simulink model "quadruped"  (R2019b)
settings: Solver=ode23t  StartTime=0.0  StopTime=Ts  RelTol=1e-3
values from neighbouring files (symbols this model uses):
  isdone = Isdone    [RL_reward.m]
  plane = [5, 50, 0.03]    [quadruped_sim_param.m]
  reward = Reward    [RL_reward.m]
  robot = Robot    [quadruped_sim_param.m]
undefined symbols (not defined in the file or in its folder): X, Y, Z
libraries: sm_lib x166, nesl_utility x90, simulink x33, rllib x1
(part 4 of 6)

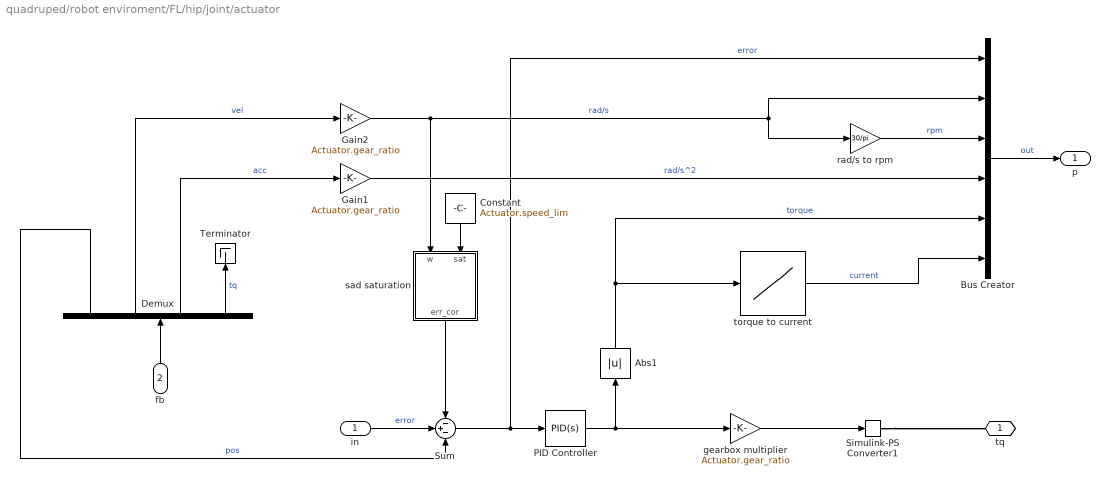
== system quadruped/robot enviroment/FL/hip/joint/actuator ==
  in : Inport
  fb : Inport  Port=2
  Abs1 : Abs
  Bus Creator : BusCreator  Inputs=6
  Constant : Constant  Value=Actuator.speed_lim
  Demux : Demux
  Gain1 : Gain  Gain=Actuator.gear_ratio
  Gain2 : Gain  Gain=Actuator.gear_ratio
  PID Controller : simulink/Continuous/PID Controller  Controller=PID  Form=Ideal  TimeDomain=Continuous-time  SampleTime=-1  IntegratorMethod=Forward Euler  FilterMethod=Forward Euler  ControllerParametersSource=internal  P=Actuator.Kp * pi / 180  I=Actuator.Ki  D=Actuator.Kd  UseFilter=on  N=Actuator.N  TunerSelectOption=Transfer Function Based (PID Tuner App)  InitialConditionSource=internal  InitialConditionForIntegrator=0  InitialConditionForFilter=0  DifferentiatorICPrevScaledInput=0  ExternalReset=none  TrackingMode=off  Kt=1  LimitOutput=on  UpperSaturationLimit=Actuator.torque_lim  LowerSaturationLimit=-Actuator.torque_lim  LinearizeAsGain=on  AntiWindupMode=none  Kb=1  POutMin=[]  POutMax=[]  IOutMin=[]  IOutMax=[]  DOutMin=[]  DOutMax=[]  NOutMin=[]  NOutMax=[]  SumOutMin=[]  SumOutMax=[]  SaturationOutMin=[]  SaturationOutMax=[]  PParamMin=[]  PParamMax=[]  IParamMin=[]  IParamMax=[]  DParamMin=[]  DParamMax=[]  NParamMin=[]  NParamMax=[]  KbParamMin=[]  KbParamMax=[]  KtParamMin=[]  KtParamMax=[]  KbOutMin=[]  KbOutMax=[]  KtOutMin=[]  KtOutMax=[]  IntegratorOutMin=[]  IntegratorOutMax=[]  FilterOutMin=[]  FilterOutMax=[]  SumI1OutMin=[]  SumI1OutMax=[]  SumI2OutMin=[]  SumI2OutMax=[]  SumI3OutMin=[]  SumI3OutMax=[]  SumI4OutMin=[]  SumI4OutMax=[]  SumDOutMin=[]  SumDOutMax=[]  DifferentiatorOutMin=[]  DifferentiatorOutMax=[]  FilterDiffOutCoefMin=[]  FilterDiffOutCoefMax=[]  ReciprocalOutMin=[]  ReciprocalOutMax=[]  SumDenOutMin=[]  SumDenOutMax=[]  SumNumOutMin=[]  SumNumOutMax=[]  DivideOutMin=[]  DivideOutMax=[]  IntegratorContinuousStateAttributes=''  IntegratorStateMustResolveToSignalObject=off  IntegratorRTWStateStorageClass=Auto  FilterContinuousStateAttributes=''  FilterStateMustResolveToSignalObject=off  FilterRTWStateStorageClass=Auto  ParallelPVariant=Passthrough  IdealPVariant=InternalParameters  IVariant=InternalParameters  DVariant=InternalParameters  IntegratorVariant=Continuous  SatVariant=Enabled  AWVariant=Passthrough  PCopyVariant=Disabled  TRVariant=Disabled  FdbkBlocksVariant=Forward  IdealPFdbkVariant=Disabled  SatFdbkVariant=Disabled  DerivativeFilterVariant=ContFilter  NVariant=InternalParameters  NCopyVariant=Disabled  FilterICVariant=InternalICsFilter  IntegratorICVariant=InternalICs  ExternalResetVariant=Disabled  TRSumVariant=Passthrough  SumFdbkVariant=Disabled  SumVariant=Sum_PID
  Simulink-PS Converter1 : nesl_utility/Simulink-PS Converter  PhysicalDomain=network_engine_domain  SubClassName=ps_input  LeftPortType=input  RightPortType=output  PseudoPeriodic=off  Frequencies=[]  NoiseDistribution=none  NoiseParameters=[]  Unit=N*m  AffineConversion=off  FilteringAndDerivatives=provide  SimscapeFilterOrder=1  InputFilterTimeConstant=0.001  UdotUserProvided=0
  Sum : Sum  Inputs=-+-
  Terminator : Terminator
  gearbox multiplier : Gain  Gain=Actuator.gear_ratio
  rad/s to rpm : Gain  Gain=30/pi
  sad saturation : Subsystem
  torque to current : Lookup_n-D  NumberOfTableDimensions=1  BreakpointsForDimension1=Actuator.torque_to_current(1,:)  Table=Actuator.torque_to_current(2,:)  InternalRulePriority=Speed  RndMeth=Simplest  InputSameDT=on
  tq : PMIOPort  Side=Right
  p : Outport
  wires:
  rad/s to rpm/1 -> Bus Creator/3  "rpm"
  Bus Creator/1 -> p/1  "out"
  torque to current/1 -> Bus Creator/6  "current"
  Sum/1 -> PID Controller/1, Bus Creator/1  "error"
  in/1 -> Sum/2  "error"
  Abs1/1 -> Bus Creator/5, torque to current/1  "torque"
  PID Controller/1 -> gearbox multiplier/1, Abs1/1
  gearbox multiplier/1 -> Simulink-PS Converter1/1
  Gain2/1 -> rad/s to rpm/1, Bus Creator/2, sad saturation/1(w)  "rad/s"
  fb/1 -> Demux/1
  Demux/1 -> Sum/3  "pos"
  Demux/2 -> Gain2/1  "vel"
  Demux/3 -> Gain1/1  "acc"
  Demux/4 -> Terminator/1  "tq"
  Gain1/1 -> Bus Creator/4  "rad/s^2"
  sad saturation/1(err_cor) -> Sum/1
  Constant/1 -> sad saturation/2(sat)
  connections:
  Simulink-PS Converter1/RConn1 -- tq/RConn1

== system quadruped/robot enviroment/FL/hip/joint/motor inertia ==
  Common Gear Constraint : sm_lib/Gears and Couplings/Gears/Common Gear Constraint  GearType=External  SpecificationType=CenterDistanceRatio  CenterDistance=0.5  CenterDistanceUnits=mm  GearRatio=Joint.actuator.gear_ratio  BaseGearRadius=10.0  BaseGearRadiusUnits=cm  FollGearRadius=10.0  FollGearRadiusUnits=cm  AssemblyGearRotation=Free
      settings: SourceProductName=Simscape Multibody  SourceProductBaseCode=MS
  Cylindrical Solid : sm_lib/Body Elements/Cylindrical Solid  GraphicAmbientColor=[0.15 0.15 0.15 1.0]  BasedOnType=Density  CenterOfMass=[0 0 0]  CenterOfMassUnits=m  GraphicDiffuseColor=[0.5 0.5 0.5]  CylinderLength=0.01  CylinderLengthUnits=m  CylinderRadius=0.01  CylinderRadiusUnits=m  Density=1000  DensityUnits=kg/m^3  DoExposeReferenceFrame=on  GraphicEmissiveColor=[0.0 0.0 0.0 1.0]  ExportEntireGeometry=off  SerializedFrames=<Frames/>  MarkerShape=Sphere  MarkerSize=10  GraphicType=FromGeometry  InertiaType=Custom  Mass=0  MassUnits=kg  MomentsOfInertia=[0 0 Joint.actuator.motor_inertia]  MomentsOfInertiaUnits=g*cm^2  GraphicOpacity=0  ProductsOfInertia=[0 0 0]  ProductsOfInertiaUnits=kg*m^2  GraphicShininess=75  GraphicSpecularColor=[0.5 0.5 0.5 1.0]  GraphicVisPropType=SimpleVisualProperties
  Revolute Joint1 : sm_lib/Joints/Revolute Joint  JointMode=Normal  SenseConstraintForce=off  SenseConstraintForceX=off  SenseConstraintForceY=off  SenseConstraintForceZ=off  SenseConstraintTorque=off  SenseConstraintTorqueX=off  SenseConstraintTorqueY=off  SenseConstraintTorqueZ=off  SenseTotalForce=off  SenseTotalForceX=off  SenseTotalForceY=off  SenseTotalForceZ=off  SenseTotalTorque=off  SenseTotalTorqueX=off  SenseTotalTorqueY=off  SenseTotalTorqueZ=off  CompositeWrenchDir=FollowerOnBase  CompositeWrenchFrame=BaseFrame  EquilibriumPosition=0  EquilibriumPositionUnits=deg  SpringStiffness=0  SpringStiffnessUnits=N*m/deg  DampingCoefficient=0  DampingCoefficientUnits=N*m/(deg/s)  TorqueActuationMode=NoTorque  MotionActuationMode=ComputedMotion  SensePosition=off  SenseVelocity=off  SenseAcceleration=off  SenseTorqueForce=off  SenseLowerLimitTorqueForce=off  SenseUpperLimitTorqueForce=off  LowerLimitSpecify=off  LowerLimitBound=-90  LowerLimitBoundUnits=deg  LowerLimitStiffness=1e4  LowerLimitStiffnessUnits=N*m/deg  LowerLimitDamping=10  LowerLimitDampingUnits=N*m/(deg/s)  LowerLimitTransitionRegionWidth=0.1  LowerLimitTransitionRegionWidthUnits=deg  UpperLimitSpecify=off  UpperLimitBound=90  UpperLimitBoundUnits=deg  UpperLimitStiffness=1e4  UpperLimitStiffnessUnits=N*m/deg  UpperLimitDamping=10  UpperLimitDampingUnits=N*m/(deg/s)  UpperLimitTransitionRegionWidth=0.1  UpperLimitTransitionRegionWidthUnits=deg  PositionTargetSpecify=off  PositionTargetPriority=High  PositionTargetValue=0  PositionTargetValueUnits=deg  VelocityTargetSpecify=off  VelocityTargetPriority=High  VelocityTargetValue=0  VelocityTargetValueUnits=deg/s
  Rigid Transform : sm_lib/Frames and Transforms/Rigid Transform  TranslationMethod=StandardAxis  TranslationStandardOffset=0.5  TranslationLengthUnit=mm  TranslationStandardAxis=+X  TranslationCartesianOffset=[0 0 0]  TranslationROffset=0  TranslationROffsetUnits=m  TranslationZOffset=0  TranslationZOffsetUnits=m  TranslationThetaOffset=0  TranslationThetaOffsetUnits=deg  RotationMethod=None  RotationAngleUnits=deg  RotationStandardAxis=+Z  RotationAngle=0.0  RotationArbitraryAxis=[0 0 1]  FollAlignAxisA=+X  BaseAlignAxisA=+Y  FollAlignAxisB=+Y  BaseAlignAxisB=+Z  RotationSequenceAxes=FollowerAxes  RotationSequence=XYX  RotationSequenceAngles=[0 0 0]  RotationSequenceAnglesUnits=deg  RotationMatrix=[1 0 0; 0 1 0; 0 0 1]
  B : PMIOPort  Side=Right
  F : PMIOPort  Port=2  Side=Left
  connections:
  Revolute Joint1/LConn1 -- Cylindrical Solid/RConn1 -- Common Gear Constraint/LConn1
  Rigid Transform/LConn1 -- Revolute Joint1/RConn1
  Common Gear Constraint/RConn1 -- F/RConn1
  B/RConn1 -- Rigid Transform/RConn1

== system quadruped/robot enviroment/FL/leg/lower joint/joint ==
  in : Inport
  Abs1 : Abs
  Bus Creator1 : BusCreator  Inputs=4
  Bus Creator2 : BusCreator  Inputs=3
  "Hip joint " : sm_lib/Joints/Revolute Joint  JointMode=Normal  SenseConstraintForce=off  SenseConstraintForceX=off  SenseConstraintForceY=off  SenseConstraintForceZ=off  SenseConstraintTorque=off  SenseConstraintTorqueX=off  SenseConstraintTorqueY=off  SenseConstraintTorqueZ=off  SenseTotalForce=off  SenseTotalForceX=off  SenseTotalForceY=off  SenseTotalForceZ=off  SenseTotalTorque=off  SenseTotalTorqueX=off  SenseTotalTorqueY=off  SenseTotalTorqueZ=off  CompositeWrenchDir=FollowerOnBase  CompositeWrenchFrame=BaseFrame  EquilibriumPosition=0  EquilibriumPositionUnits=rad  SpringStiffness=Joint.stiffness  SpringStiffnessUnits=N*m/deg  DampingCoefficient=Joint.damping  DampingCoefficientUnits=N*m/(deg/s)  TorqueActuationMode=InputTorque  MotionActuationMode=ComputedMotion  SensePosition=on  SenseVelocity=on  SenseAcceleration=on  SenseTorqueForce=on  SenseLowerLimitTorqueForce=off  SenseUpperLimitTorqueForce=off  LowerLimitSpecify=off  LowerLimitBound=-90  LowerLimitBoundUnits=deg  LowerLimitStiffness=1e4  LowerLimitStiffnessUnits=N*m/deg  LowerLimitDamping=10  LowerLimitDampingUnits=N*m/(deg/s)  LowerLimitTransitionRegionWidth=0.1  LowerLimitTransitionRegionWidthUnits=deg  UpperLimitSpecify=off  UpperLimitBound=90  UpperLimitBoundUnits=deg  UpperLimitStiffness=1e4  UpperLimitStiffnessUnits=N*m/deg  UpperLimitDamping=10  UpperLimitDampingUnits=N*m/(deg/s)  UpperLimitTransitionRegionWidth=0.1  UpperLimitTransitionRegionWidthUnits=deg  PositionTargetSpecify=on  PositionTargetPriority=High  PositionTargetValue=Joint.base_angle  PositionTargetValueUnits=rad  VelocityTargetSpecify=off  VelocityTargetPriority=High  VelocityTargetValue=0  VelocityTargetValueUnits=deg/s
  PS-Simulink Converter{3..6} (4 alike) : nesl_utility/PS-Simulink Converter  PhysicalDomain=network_engine_domain  SubClassName=ps_output  LeftPortType=input  RightPortType=output  PseudoPeriodic=off  Frequencies=[]  Unit=inherit  AffineConversion=off
  actuator : Subsystem  mask{Actuator=Joint.actuator}
  motor inertia : Subsystem
  B : PMIOPort  Side=Left
  F : PMIOPort  Port=2  Side=Right
  p : Outport
  wires:
  PS-Simulink Converter5/1 -> Bus Creator1/3  "b"
  PS-Simulink Converter6/1 -> Abs1/1, Bus Creator1/4  "t"
  PS-Simulink Converter3/1 -> Bus Creator1/2  "w"
  in/1 -> actuator/1(in)
  Bus Creator1/1 -> actuator/2(fb)
  actuator/1(p) -> Bus Creator2/3  "actuator"
  Bus Creator2/1 -> p/1
  Abs1/1 -> Bus Creator2/2  "joint torque"
  PS-Simulink Converter4/1 -> Bus Creator2/1, Bus Creator1/1  "position"
  connections:
  "Hip joint "/RConn4 -- PS-Simulink Converter5/LConn1
  motor inertia/RConn1 -- "Hip joint "/LConn1 -- B/RConn1
  actuator/RConn1 -- "Hip joint "/LConn2
  "Hip joint "/RConn5 -- PS-Simulink Converter6/LConn1
  "Hip joint "/RConn2 -- PS-Simulink Converter4/LConn1
  "Hip joint "/RConn1 -- motor inertia/LConn1 -- F/RConn1
  "Hip joint "/RConn3 -- PS-Simulink Converter3/LConn1

== system quadruped/robot enviroment/FL/leg/upper joint/joint ==
  in : Inport
  Abs1 : Abs
  Bus Creator1 : BusCreator  Inputs=4
  Bus Creator2 : BusCreator  Inputs=3
  "Hip joint " : sm_lib/Joints/Revolute Joint  JointMode=Normal  SenseConstraintForce=off  SenseConstraintForceX=off  SenseConstraintForceY=off  SenseConstraintForceZ=off  SenseConstraintTorque=off  SenseConstraintTorqueX=off  SenseConstraintTorqueY=off  SenseConstraintTorqueZ=off  SenseTotalForce=off  SenseTotalForceX=off  SenseTotalForceY=off  SenseTotalForceZ=off  SenseTotalTorque=off  SenseTotalTorqueX=off  SenseTotalTorqueY=off  SenseTotalTorqueZ=off  CompositeWrenchDir=FollowerOnBase  CompositeWrenchFrame=BaseFrame  EquilibriumPosition=0  EquilibriumPositionUnits=rad  SpringStiffness=Joint.stiffness  SpringStiffnessUnits=N*m/deg  DampingCoefficient=Joint.damping  DampingCoefficientUnits=N*m/(deg/s)  TorqueActuationMode=InputTorque  MotionActuationMode=ComputedMotion  SensePosition=on  SenseVelocity=on  SenseAcceleration=on  SenseTorqueForce=on  SenseLowerLimitTorqueForce=off  SenseUpperLimitTorqueForce=off  LowerLimitSpecify=off  LowerLimitBound=-90  LowerLimitBoundUnits=deg  LowerLimitStiffness=1e4  LowerLimitStiffnessUnits=N*m/deg  LowerLimitDamping=10  LowerLimitDampingUnits=N*m/(deg/s)  LowerLimitTransitionRegionWidth=0.1  LowerLimitTransitionRegionWidthUnits=deg  UpperLimitSpecify=off  UpperLimitBound=90  UpperLimitBoundUnits=deg  UpperLimitStiffness=1e4  UpperLimitStiffnessUnits=N*m/deg  UpperLimitDamping=10  UpperLimitDampingUnits=N*m/(deg/s)  UpperLimitTransitionRegionWidth=0.1  UpperLimitTransitionRegionWidthUnits=deg  PositionTargetSpecify=on  PositionTargetPriority=High  PositionTargetValue=Joint.base_angle  PositionTargetValueUnits=rad  VelocityTargetSpecify=off  VelocityTargetPriority=High  VelocityTargetValue=0  VelocityTargetValueUnits=deg/s
  PS-Simulink Converter{3..6} (4 alike) : nesl_utility/PS-Simulink Converter  PhysicalDomain=network_engine_domain  SubClassName=ps_output  LeftPortType=input  RightPortType=output  PseudoPeriodic=off  Frequencies=[]  Unit=inherit  AffineConversion=off
  actuator : Subsystem  mask{Actuator=Joint.actuator}
  motor inertia : Subsystem
  B : PMIOPort  Side=Left
  F : PMIOPort  Port=2  Side=Right
  p : Outport
  wires:
  PS-Simulink Converter5/1 -> Bus Creator1/3  "b"
  PS-Simulink Converter6/1 -> Abs1/1, Bus Creator1/4  "t"
  PS-Simulink Converter3/1 -> Bus Creator1/2  "w"
  in/1 -> actuator/1(in)
  Bus Creator1/1 -> actuator/2(fb)
  actuator/1(p) -> Bus Creator2/3  "actuator"
  Bus Creator2/1 -> p/1
  Abs1/1 -> Bus Creator2/2  "joint torque"
  PS-Simulink Converter4/1 -> Bus Creator2/1, Bus Creator1/1  "position"
  connections:
  "Hip joint "/RConn4 -- PS-Simulink Converter5/LConn1
  motor inertia/RConn1 -- "Hip joint "/LConn1 -- B/RConn1
  actuator/RConn1 -- "Hip joint "/LConn2
  "Hip joint "/RConn5 -- PS-Simulink Converter6/LConn1
  "Hip joint "/RConn2 -- PS-Simulink Converter4/LConn1
  "Hip joint "/RConn1 -- motor inertia/LConn1 -- F/RConn1
  "Hip joint "/RConn3 -- PS-Simulink Converter3/LConn1

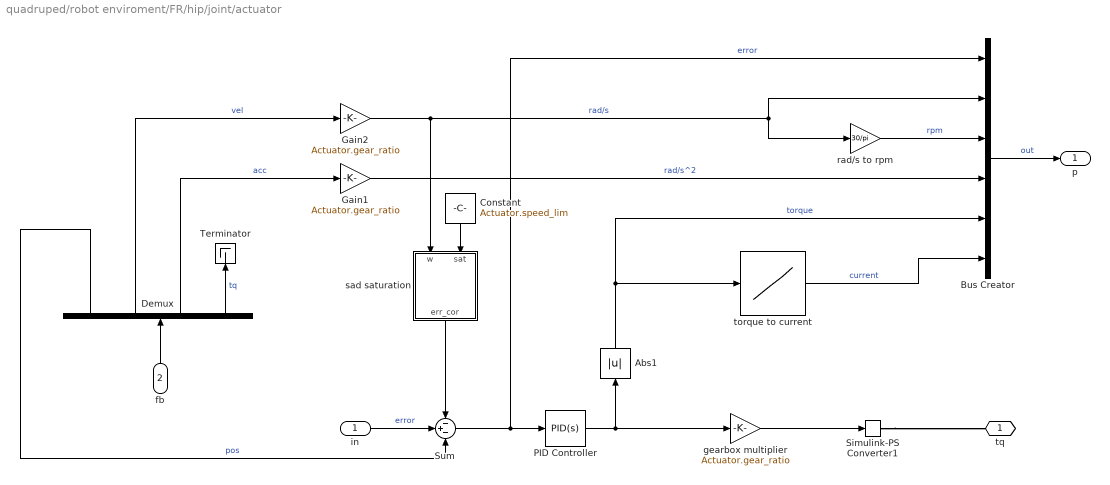
== system quadruped/robot enviroment/FR/hip/joint/actuator ==
  in : Inport
  fb : Inport  Port=2
  Abs1 : Abs
  Bus Creator : BusCreator  Inputs=6
  Constant : Constant  Value=Actuator.speed_lim
  Demux : Demux
  Gain1 : Gain  Gain=Actuator.gear_ratio
  Gain2 : Gain  Gain=Actuator.gear_ratio
  PID Controller : simulink/Continuous/PID Controller  Controller=PID  Form=Ideal  TimeDomain=Continuous-time  SampleTime=-1  IntegratorMethod=Forward Euler  FilterMethod=Forward Euler  ControllerParametersSource=internal  P=Actuator.Kp * pi / 180  I=Actuator.Ki  D=Actuator.Kd  UseFilter=on  N=Actuator.N  TunerSelectOption=Transfer Function Based (PID Tuner App)  InitialConditionSource=internal  InitialConditionForIntegrator=0  InitialConditionForFilter=0  DifferentiatorICPrevScaledInput=0  ExternalReset=none  TrackingMode=off  Kt=1  LimitOutput=on  UpperSaturationLimit=Actuator.torque_lim  LowerSaturationLimit=-Actuator.torque_lim  LinearizeAsGain=on  AntiWindupMode=none  Kb=1  POutMin=[]  POutMax=[]  IOutMin=[]  IOutMax=[]  DOutMin=[]  DOutMax=[]  NOutMin=[]  NOutMax=[]  SumOutMin=[]  SumOutMax=[]  SaturationOutMin=[]  SaturationOutMax=[]  PParamMin=[]  PParamMax=[]  IParamMin=[]  IParamMax=[]  DParamMin=[]  DParamMax=[]  NParamMin=[]  NParamMax=[]  KbParamMin=[]  KbParamMax=[]  KtParamMin=[]  KtParamMax=[]  KbOutMin=[]  KbOutMax=[]  KtOutMin=[]  KtOutMax=[]  IntegratorOutMin=[]  IntegratorOutMax=[]  FilterOutMin=[]  FilterOutMax=[]  SumI1OutMin=[]  SumI1OutMax=[]  SumI2OutMin=[]  SumI2OutMax=[]  SumI3OutMin=[]  SumI3OutMax=[]  SumI4OutMin=[]  SumI4OutMax=[]  SumDOutMin=[]  SumDOutMax=[]  DifferentiatorOutMin=[]  DifferentiatorOutMax=[]  FilterDiffOutCoefMin=[]  FilterDiffOutCoefMax=[]  ReciprocalOutMin=[]  ReciprocalOutMax=[]  SumDenOutMin=[]  SumDenOutMax=[]  SumNumOutMin=[]  SumNumOutMax=[]  DivideOutMin=[]  DivideOutMax=[]  IntegratorContinuousStateAttributes=''  IntegratorStateMustResolveToSignalObject=off  IntegratorRTWStateStorageClass=Auto  FilterContinuousStateAttributes=''  FilterStateMustResolveToSignalObject=off  FilterRTWStateStorageClass=Auto  ParallelPVariant=Passthrough  IdealPVariant=InternalParameters  IVariant=InternalParameters  DVariant=InternalParameters  IntegratorVariant=Continuous  SatVariant=Enabled  AWVariant=Passthrough  PCopyVariant=Disabled  TRVariant=Disabled  FdbkBlocksVariant=Forward  IdealPFdbkVariant=Disabled  SatFdbkVariant=Disabled  DerivativeFilterVariant=ContFilter  NVariant=InternalParameters  NCopyVariant=Disabled  FilterICVariant=InternalICsFilter  IntegratorICVariant=InternalICs  ExternalResetVariant=Disabled  TRSumVariant=Passthrough  SumFdbkVariant=Disabled  SumVariant=Sum_PID
  Simulink-PS Converter1 : nesl_utility/Simulink-PS Converter  PhysicalDomain=network_engine_domain  SubClassName=ps_input  LeftPortType=input  RightPortType=output  PseudoPeriodic=off  Frequencies=[]  NoiseDistribution=none  NoiseParameters=[]  Unit=N*m  AffineConversion=off  FilteringAndDerivatives=provide  SimscapeFilterOrder=1  InputFilterTimeConstant=0.001  UdotUserProvided=0
  Sum : Sum  Inputs=-+-
  Terminator : Terminator
  gearbox multiplier : Gain  Gain=Actuator.gear_ratio
  rad/s to rpm : Gain  Gain=30/pi
  sad saturation : Subsystem
  torque to current : Lookup_n-D  NumberOfTableDimensions=1  BreakpointsForDimension1=Actuator.torque_to_current(1,:)  Table=Actuator.torque_to_current(2,:)  InternalRulePriority=Speed  RndMeth=Simplest  InputSameDT=on
  tq : PMIOPort  Side=Right
  p : Outport
  wires:
  rad/s to rpm/1 -> Bus Creator/3  "rpm"
  Bus Creator/1 -> p/1  "out"
  torque to current/1 -> Bus Creator/6  "current"
  Sum/1 -> PID Controller/1, Bus Creator/1  "error"
  in/1 -> Sum/2  "error"
  Abs1/1 -> Bus Creator/5, torque to current/1  "torque"
  PID Controller/1 -> gearbox multiplier/1, Abs1/1
  gearbox multiplier/1 -> Simulink-PS Converter1/1
  Gain2/1 -> rad/s to rpm/1, Bus Creator/2, sad saturation/1(w)  "rad/s"
  fb/1 -> Demux/1
  Demux/1 -> Sum/3  "pos"
  Demux/2 -> Gain2/1  "vel"
  Demux/3 -> Gain1/1  "acc"
  Demux/4 -> Terminator/1  "tq"
  Gain1/1 -> Bus Creator/4  "rad/s^2"
  sad saturation/1(err_cor) -> Sum/1
  Constant/1 -> sad saturation/2(sat)
  connections:
  Simulink-PS Converter1/RConn1 -- tq/RConn1

== system quadruped/robot enviroment/FR/hip/joint/motor inertia ==
  Common Gear Constraint : sm_lib/Gears and Couplings/Gears/Common Gear Constraint  GearType=External  SpecificationType=CenterDistanceRatio  CenterDistance=0.5  CenterDistanceUnits=mm  GearRatio=Joint.actuator.gear_ratio  BaseGearRadius=10.0  BaseGearRadiusUnits=cm  FollGearRadius=10.0  FollGearRadiusUnits=cm  AssemblyGearRotation=Free
      settings: SourceProductName=Simscape Multibody  SourceProductBaseCode=MS
  Cylindrical Solid : sm_lib/Body Elements/Cylindrical Solid  GraphicAmbientColor=[0.15 0.15 0.15 1.0]  BasedOnType=Density  CenterOfMass=[0 0 0]  CenterOfMassUnits=m  GraphicDiffuseColor=[0.5 0.5 0.5]  CylinderLength=0.01  CylinderLengthUnits=m  CylinderRadius=0.01  CylinderRadiusUnits=m  Density=1000  DensityUnits=kg/m^3  DoExposeReferenceFrame=on  GraphicEmissiveColor=[0.0 0.0 0.0 1.0]  ExportEntireGeometry=off  SerializedFrames=<Frames/>  MarkerShape=Sphere  MarkerSize=10  GraphicType=FromGeometry  InertiaType=Custom  Mass=0  MassUnits=kg  MomentsOfInertia=[0 0 Joint.actuator.motor_inertia]  MomentsOfInertiaUnits=g*cm^2  GraphicOpacity=0  ProductsOfInertia=[0 0 0]  ProductsOfInertiaUnits=kg*m^2  GraphicShininess=75  GraphicSpecularColor=[0.5 0.5 0.5 1.0]  GraphicVisPropType=SimpleVisualProperties
  Revolute Joint1 : sm_lib/Joints/Revolute Joint  JointMode=Normal  SenseConstraintForce=off  SenseConstraintForceX=off  SenseConstraintForceY=off  SenseConstraintForceZ=off  SenseConstraintTorque=off  SenseConstraintTorqueX=off  SenseConstraintTorqueY=off  SenseConstraintTorqueZ=off  SenseTotalForce=off  SenseTotalForceX=off  SenseTotalForceY=off  SenseTotalForceZ=off  SenseTotalTorque=off  SenseTotalTorqueX=off  SenseTotalTorqueY=off  SenseTotalTorqueZ=off  CompositeWrenchDir=FollowerOnBase  CompositeWrenchFrame=BaseFrame  EquilibriumPosition=0  EquilibriumPositionUnits=deg  SpringStiffness=0  SpringStiffnessUnits=N*m/deg  DampingCoefficient=0  DampingCoefficientUnits=N*m/(deg/s)  TorqueActuationMode=NoTorque  MotionActuationMode=ComputedMotion  SensePosition=off  SenseVelocity=off  SenseAcceleration=off  SenseTorqueForce=off  SenseLowerLimitTorqueForce=off  SenseUpperLimitTorqueForce=off  LowerLimitSpecify=off  LowerLimitBound=-90  LowerLimitBoundUnits=deg  LowerLimitStiffness=1e4  LowerLimitStiffnessUnits=N*m/deg  LowerLimitDamping=10  LowerLimitDampingUnits=N*m/(deg/s)  LowerLimitTransitionRegionWidth=0.1  LowerLimitTransitionRegionWidthUnits=deg  UpperLimitSpecify=off  UpperLimitBound=90  UpperLimitBoundUnits=deg  UpperLimitStiffness=1e4  UpperLimitStiffnessUnits=N*m/deg  UpperLimitDamping=10  UpperLimitDampingUnits=N*m/(deg/s)  UpperLimitTransitionRegionWidth=0.1  UpperLimitTransitionRegionWidthUnits=deg  PositionTargetSpecify=off  PositionTargetPriority=High  PositionTargetValue=0  PositionTargetValueUnits=deg  VelocityTargetSpecify=off  VelocityTargetPriority=High  VelocityTargetValue=0  VelocityTargetValueUnits=deg/s
  Rigid Transform : sm_lib/Frames and Transforms/Rigid Transform  TranslationMethod=StandardAxis  TranslationStandardOffset=0.5  TranslationLengthUnit=mm  TranslationStandardAxis=+X  TranslationCartesianOffset=[0 0 0]  TranslationROffset=0  TranslationROffsetUnits=m  TranslationZOffset=0  TranslationZOffsetUnits=m  TranslationThetaOffset=0  TranslationThetaOffsetUnits=deg  RotationMethod=None  RotationAngleUnits=deg  RotationStandardAxis=+Z  RotationAngle=0.0  RotationArbitraryAxis=[0 0 1]  FollAlignAxisA=+X  BaseAlignAxisA=+Y  FollAlignAxisB=+Y  BaseAlignAxisB=+Z  RotationSequenceAxes=FollowerAxes  RotationSequence=XYX  RotationSequenceAngles=[0 0 0]  RotationSequenceAnglesUnits=deg  RotationMatrix=[1 0 0; 0 1 0; 0 0 1]
  B : PMIOPort  Side=Right
  F : PMIOPort  Port=2  Side=Left
  connections:
  Revolute Joint1/LConn1 -- Cylindrical Solid/RConn1 -- Common Gear Constraint/LConn1
  Rigid Transform/LConn1 -- Revolute Joint1/RConn1
  Common Gear Constraint/RConn1 -- F/RConn1
  B/RConn1 -- Rigid Transform/RConn1

== system quadruped/robot enviroment/FR/leg/lower joint/joint ==
  in : Inport
  Abs1 : Abs
  Bus Creator1 : BusCreator  Inputs=4
  Bus Creator2 : BusCreator  Inputs=3
  "Hip joint " : sm_lib/Joints/Revolute Joint  JointMode=Normal  SenseConstraintForce=off  SenseConstraintForceX=off  SenseConstraintForceY=off  SenseConstraintForceZ=off  SenseConstraintTorque=off  SenseConstraintTorqueX=off  SenseConstraintTorqueY=off  SenseConstraintTorqueZ=off  SenseTotalForce=off  SenseTotalForceX=off  SenseTotalForceY=off  SenseTotalForceZ=off  SenseTotalTorque=off  SenseTotalTorqueX=off  SenseTotalTorqueY=off  SenseTotalTorqueZ=off  CompositeWrenchDir=FollowerOnBase  CompositeWrenchFrame=BaseFrame  EquilibriumPosition=0  EquilibriumPositionUnits=rad  SpringStiffness=Joint.stiffness  SpringStiffnessUnits=N*m/deg  DampingCoefficient=Joint.damping  DampingCoefficientUnits=N*m/(deg/s)  TorqueActuationMode=InputTorque  MotionActuationMode=ComputedMotion  SensePosition=on  SenseVelocity=on  SenseAcceleration=on  SenseTorqueForce=on  SenseLowerLimitTorqueForce=off  SenseUpperLimitTorqueForce=off  LowerLimitSpecify=off  LowerLimitBound=-90  LowerLimitBoundUnits=deg  LowerLimitStiffness=1e4  LowerLimitStiffnessUnits=N*m/deg  LowerLimitDamping=10  LowerLimitDampingUnits=N*m/(deg/s)  LowerLimitTransitionRegionWidth=0.1  LowerLimitTransitionRegionWidthUnits=deg  UpperLimitSpecify=off  UpperLimitBound=90  UpperLimitBoundUnits=deg  UpperLimitStiffness=1e4  UpperLimitStiffnessUnits=N*m/deg  UpperLimitDamping=10  UpperLimitDampingUnits=N*m/(deg/s)  UpperLimitTransitionRegionWidth=0.1  UpperLimitTransitionRegionWidthUnits=deg  PositionTargetSpecify=on  PositionTargetPriority=High  PositionTargetValue=Joint.base_angle  PositionTargetValueUnits=rad  VelocityTargetSpecify=off  VelocityTargetPriority=High  VelocityTargetValue=0  VelocityTargetValueUnits=deg/s
  PS-Simulink Converter{3..6} (4 alike) : nesl_utility/PS-Simulink Converter  PhysicalDomain=network_engine_domain  SubClassName=ps_output  LeftPortType=input  RightPortType=output  PseudoPeriodic=off  Frequencies=[]  Unit=inherit  AffineConversion=off
  actuator : Subsystem  mask{Actuator=Joint.actuator}
  motor inertia : Subsystem
  B : PMIOPort  Side=Left
  F : PMIOPort  Port=2  Side=Right
  p : Outport
  wires:
  PS-Simulink Converter5/1 -> Bus Creator1/3  "b"
  PS-Simulink Converter6/1 -> Abs1/1, Bus Creator1/4  "t"
  PS-Simulink Converter3/1 -> Bus Creator1/2  "w"
  in/1 -> actuator/1(in)
  Bus Creator1/1 -> actuator/2(fb)
  actuator/1(p) -> Bus Creator2/3  "actuator"
  Bus Creator2/1 -> p/1
  Abs1/1 -> Bus Creator2/2  "joint torque"
  PS-Simulink Converter4/1 -> Bus Creator2/1, Bus Creator1/1  "position"
  connections:
  "Hip joint "/RConn4 -- PS-Simulink Converter5/LConn1
  motor inertia/RConn1 -- "Hip joint "/LConn1 -- B/RConn1
  actuator/RConn1 -- "Hip joint "/LConn2
  "Hip joint "/RConn5 -- PS-Simulink Converter6/LConn1
  "Hip joint "/RConn2 -- PS-Simulink Converter4/LConn1
  "Hip joint "/RConn1 -- motor inertia/LConn1 -- F/RConn1
  "Hip joint "/RConn3 -- PS-Simulink Converter3/LConn1

== system quadruped/robot enviroment/FR/leg/upper joint/joint ==
  in : Inport
  Abs1 : Abs
  Bus Creator1 : BusCreator  Inputs=4
  Bus Creator2 : BusCreator  Inputs=3
  "Hip joint " : sm_lib/Joints/Revolute Joint  JointMode=Normal  SenseConstraintForce=off  SenseConstraintForceX=off  SenseConstraintForceY=off  SenseConstraintForceZ=off  SenseConstraintTorque=off  SenseConstraintTorqueX=off  SenseConstraintTorqueY=off  SenseConstraintTorqueZ=off  SenseTotalForce=off  SenseTotalForceX=off  SenseTotalForceY=off  SenseTotalForceZ=off  SenseTotalTorque=off  SenseTotalTorqueX=off  SenseTotalTorqueY=off  SenseTotalTorqueZ=off  CompositeWrenchDir=FollowerOnBase  CompositeWrenchFrame=BaseFrame  EquilibriumPosition=0  EquilibriumPositionUnits=rad  SpringStiffness=Joint.stiffness  SpringStiffnessUnits=N*m/deg  DampingCoefficient=Joint.damping  DampingCoefficientUnits=N*m/(deg/s)  TorqueActuationMode=InputTorque  MotionActuationMode=ComputedMotion  SensePosition=on  SenseVelocity=on  SenseAcceleration=on  SenseTorqueForce=on  SenseLowerLimitTorqueForce=off  SenseUpperLimitTorqueForce=off  LowerLimitSpecify=off  LowerLimitBound=-90  LowerLimitBoundUnits=deg  LowerLimitStiffness=1e4  LowerLimitStiffnessUnits=N*m/deg  LowerLimitDamping=10  LowerLimitDampingUnits=N*m/(deg/s)  LowerLimitTransitionRegionWidth=0.1  LowerLimitTransitionRegionWidthUnits=deg  UpperLimitSpecify=off  UpperLimitBound=90  UpperLimitBoundUnits=deg  UpperLimitStiffness=1e4  UpperLimitStiffnessUnits=N*m/deg  UpperLimitDamping=10  UpperLimitDampingUnits=N*m/(deg/s)  UpperLimitTransitionRegionWidth=0.1  UpperLimitTransitionRegionWidthUnits=deg  PositionTargetSpecify=on  PositionTargetPriority=High  PositionTargetValue=Joint.base_angle  PositionTargetValueUnits=rad  VelocityTargetSpecify=off  VelocityTargetPriority=High  VelocityTargetValue=0  VelocityTargetValueUnits=deg/s
  PS-Simulink Converter{3..6} (4 alike) : nesl_utility/PS-Simulink Converter  PhysicalDomain=network_engine_domain  SubClassName=ps_output  LeftPortType=input  RightPortType=output  PseudoPeriodic=off  Frequencies=[]  Unit=inherit  AffineConversion=off
  actuator : Subsystem  mask{Actuator=Joint.actuator}
  motor inertia : Subsystem
  B : PMIOPort  Side=Left
  F : PMIOPort  Port=2  Side=Right
  p : Outport
  wires:
  PS-Simulink Converter5/1 -> Bus Creator1/3  "b"
  PS-Simulink Converter6/1 -> Abs1/1, Bus Creator1/4  "t"
  PS-Simulink Converter3/1 -> Bus Creator1/2  "w"
  in/1 -> actuator/1(in)
  Bus Creator1/1 -> actuator/2(fb)
  actuator/1(p) -> Bus Creator2/3  "actuator"
  Bus Creator2/1 -> p/1
  Abs1/1 -> Bus Creator2/2  "joint torque"
  PS-Simulink Converter4/1 -> Bus Creator2/1, Bus Creator1/1  "position"
  connections:
  "Hip joint "/RConn4 -- PS-Simulink Converter5/LConn1
  motor inertia/RConn1 -- "Hip joint "/LConn1 -- B/RConn1
  actuator/RConn1 -- "Hip joint "/LConn2
  "Hip joint "/RConn5 -- PS-Simulink Converter6/LConn1
  "Hip joint "/RConn2 -- PS-Simulink Converter4/LConn1
  "Hip joint "/RConn1 -- motor inertia/LConn1 -- F/RConn1
  "Hip joint "/RConn3 -- PS-Simulink Converter3/LConn1

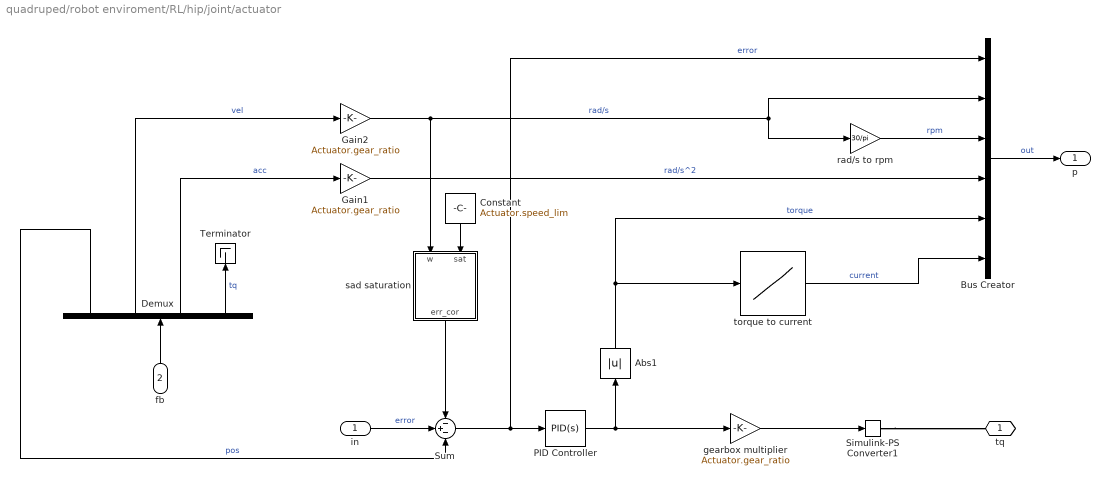
== system quadruped/robot enviroment/RL/hip/joint/actuator ==
  in : Inport
  fb : Inport  Port=2
  Abs1 : Abs
  Bus Creator : BusCreator  Inputs=6
  Constant : Constant  Value=Actuator.speed_lim
  Demux : Demux
  Gain1 : Gain  Gain=Actuator.gear_ratio
  Gain2 : Gain  Gain=Actuator.gear_ratio
  PID Controller : simulink/Continuous/PID Controller  Controller=PID  Form=Ideal  TimeDomain=Continuous-time  SampleTime=-1  IntegratorMethod=Forward Euler  FilterMethod=Forward Euler  ControllerParametersSource=internal  P=Actuator.Kp * pi / 180  I=Actuator.Ki  D=Actuator.Kd  UseFilter=on  N=Actuator.N  TunerSelectOption=Transfer Function Based (PID Tuner App)  InitialConditionSource=internal  InitialConditionForIntegrator=0  InitialConditionForFilter=0  DifferentiatorICPrevScaledInput=0  ExternalReset=none  TrackingMode=off  Kt=1  LimitOutput=on  UpperSaturationLimit=Actuator.torque_lim  LowerSaturationLimit=-Actuator.torque_lim  LinearizeAsGain=on  AntiWindupMode=none  Kb=1  POutMin=[]  POutMax=[]  IOutMin=[]  IOutMax=[]  DOutMin=[]  DOutMax=[]  NOutMin=[]  NOutMax=[]  SumOutMin=[]  SumOutMax=[]  SaturationOutMin=[]  SaturationOutMax=[]  PParamMin=[]  PParamMax=[]  IParamMin=[]  IParamMax=[]  DParamMin=[]  DParamMax=[]  NParamMin=[]  NParamMax=[]  KbParamMin=[]  KbParamMax=[]  KtParamMin=[]  KtParamMax=[]  KbOutMin=[]  KbOutMax=[]  KtOutMin=[]  KtOutMax=[]  IntegratorOutMin=[]  IntegratorOutMax=[]  FilterOutMin=[]  FilterOutMax=[]  SumI1OutMin=[]  SumI1OutMax=[]  SumI2OutMin=[]  SumI2OutMax=[]  SumI3OutMin=[]  SumI3OutMax=[]  SumI4OutMin=[]  SumI4OutMax=[]  SumDOutMin=[]  SumDOutMax=[]  DifferentiatorOutMin=[]  DifferentiatorOutMax=[]  FilterDiffOutCoefMin=[]  FilterDiffOutCoefMax=[]  ReciprocalOutMin=[]  ReciprocalOutMax=[]  SumDenOutMin=[]  SumDenOutMax=[]  SumNumOutMin=[]  SumNumOutMax=[]  DivideOutMin=[]  DivideOutMax=[]  IntegratorContinuousStateAttributes=''  IntegratorStateMustResolveToSignalObject=off  IntegratorRTWStateStorageClass=Auto  FilterContinuousStateAttributes=''  FilterStateMustResolveToSignalObject=off  FilterRTWStateStorageClass=Auto  ParallelPVariant=Passthrough  IdealPVariant=InternalParameters  IVariant=InternalParameters  DVariant=InternalParameters  IntegratorVariant=Continuous  SatVariant=Enabled  AWVariant=Passthrough  PCopyVariant=Disabled  TRVariant=Disabled  FdbkBlocksVariant=Forward  IdealPFdbkVariant=Disabled  SatFdbkVariant=Disabled  DerivativeFilterVariant=ContFilter  NVariant=InternalParameters  NCopyVariant=Disabled  FilterICVariant=InternalICsFilter  IntegratorICVariant=InternalICs  ExternalResetVariant=Disabled  TRSumVariant=Passthrough  SumFdbkVariant=Disabled  SumVariant=Sum_PID
  Simulink-PS Converter1 : nesl_utility/Simulink-PS Converter  PhysicalDomain=network_engine_domain  SubClassName=ps_input  LeftPortType=input  RightPortType=output  PseudoPeriodic=off  Frequencies=[]  NoiseDistribution=none  NoiseParameters=[]  Unit=N*m  AffineConversion=off  FilteringAndDerivatives=provide  SimscapeFilterOrder=1  InputFilterTimeConstant=0.001  UdotUserProvided=0
  Sum : Sum  Inputs=-+-
  Terminator : Terminator
  gearbox multiplier : Gain  Gain=Actuator.gear_ratio
  rad/s to rpm : Gain  Gain=30/pi
  sad saturation : Subsystem
  torque to current : Lookup_n-D  NumberOfTableDimensions=1  BreakpointsForDimension1=Actuator.torque_to_current(1,:)  Table=Actuator.torque_to_current(2,:)  InternalRulePriority=Speed  RndMeth=Simplest  InputSameDT=on
  tq : PMIOPort  Side=Right
  p : Outport
  wires:
  rad/s to rpm/1 -> Bus Creator/3  "rpm"
  Bus Creator/1 -> p/1  "out"
  torque to current/1 -> Bus Creator/6  "current"
  Sum/1 -> PID Controller/1, Bus Creator/1  "error"
  in/1 -> Sum/2  "error"
  Abs1/1 -> Bus Creator/5, torque to current/1  "torque"
  PID Controller/1 -> gearbox multiplier/1, Abs1/1
  gearbox multiplier/1 -> Simulink-PS Converter1/1
  Gain2/1 -> rad/s to rpm/1, Bus Creator/2, sad saturation/1(w)  "rad/s"
  fb/1 -> Demux/1
  Demux/1 -> Sum/3  "pos"
  Demux/2 -> Gain2/1  "vel"
  Demux/3 -> Gain1/1  "acc"
  Demux/4 -> Terminator/1  "tq"
  Gain1/1 -> Bus Creator/4  "rad/s^2"
  sad saturation/1(err_cor) -> Sum/1
  Constant/1 -> sad saturation/2(sat)
  connections:
  Simulink-PS Converter1/RConn1 -- tq/RConn1

== system quadruped/robot enviroment/RL/hip/joint/motor inertia ==
  Common Gear Constraint : sm_lib/Gears and Couplings/Gears/Common Gear Constraint  GearType=External  SpecificationType=CenterDistanceRatio  CenterDistance=0.5  CenterDistanceUnits=mm  GearRatio=Joint.actuator.gear_ratio  BaseGearRadius=10.0  BaseGearRadiusUnits=cm  FollGearRadius=10.0  FollGearRadiusUnits=cm  AssemblyGearRotation=Free
      settings: SourceProductName=Simscape Multibody  SourceProductBaseCode=MS
  Cylindrical Solid : sm_lib/Body Elements/Cylindrical Solid  GraphicAmbientColor=[0.15 0.15 0.15 1.0]  BasedOnType=Density  CenterOfMass=[0 0 0]  CenterOfMassUnits=m  GraphicDiffuseColor=[0.5 0.5 0.5]  CylinderLength=0.01  CylinderLengthUnits=m  CylinderRadius=0.01  CylinderRadiusUnits=m  Density=1000  DensityUnits=kg/m^3  DoExposeReferenceFrame=on  GraphicEmissiveColor=[0.0 0.0 0.0 1.0]  ExportEntireGeometry=off  SerializedFrames=<Frames/>  MarkerShape=Sphere  MarkerSize=10  GraphicType=FromGeometry  InertiaType=Custom  Mass=0  MassUnits=kg  MomentsOfInertia=[0 0 Joint.actuator.motor_inertia]  MomentsOfInertiaUnits=g*cm^2  GraphicOpacity=0  ProductsOfInertia=[0 0 0]  ProductsOfInertiaUnits=kg*m^2  GraphicShininess=75  GraphicSpecularColor=[0.5 0.5 0.5 1.0]  GraphicVisPropType=SimpleVisualProperties
  Revolute Joint1 : sm_lib/Joints/Revolute Joint  JointMode=Normal  SenseConstraintForce=off  SenseConstraintForceX=off  SenseConstraintForceY=off  SenseConstraintForceZ=off  SenseConstraintTorque=off  SenseConstraintTorqueX=off  SenseConstraintTorqueY=off  SenseConstraintTorqueZ=off  SenseTotalForce=off  SenseTotalForceX=off  SenseTotalForceY=off  SenseTotalForceZ=off  SenseTotalTorque=off  SenseTotalTorqueX=off  SenseTotalTorqueY=off  SenseTotalTorqueZ=off  CompositeWrenchDir=FollowerOnBase  CompositeWrenchFrame=BaseFrame  EquilibriumPosition=0  EquilibriumPositionUnits=deg  SpringStiffness=0  SpringStiffnessUnits=N*m/deg  DampingCoefficient=0  DampingCoefficientUnits=N*m/(deg/s)  TorqueActuationMode=NoTorque  MotionActuationMode=ComputedMotion  SensePosition=off  SenseVelocity=off  SenseAcceleration=off  SenseTorqueForce=off  SenseLowerLimitTorqueForce=off  SenseUpperLimitTorqueForce=off  LowerLimitSpecify=off  LowerLimitBound=-90  LowerLimitBoundUnits=deg  LowerLimitStiffness=1e4  LowerLimitStiffnessUnits=N*m/deg  LowerLimitDamping=10  LowerLimitDampingUnits=N*m/(deg/s)  LowerLimitTransitionRegionWidth=0.1  LowerLimitTransitionRegionWidthUnits=deg  UpperLimitSpecify=off  UpperLimitBound=90  UpperLimitBoundUnits=deg  UpperLimitStiffness=1e4  UpperLimitStiffnessUnits=N*m/deg  UpperLimitDamping=10  UpperLimitDampingUnits=N*m/(deg/s)  UpperLimitTransitionRegionWidth=0.1  UpperLimitTransitionRegionWidthUnits=deg  PositionTargetSpecify=off  PositionTargetPriority=High  PositionTargetValue=0  PositionTargetValueUnits=deg  VelocityTargetSpecify=off  VelocityTargetPriority=High  VelocityTargetValue=0  VelocityTargetValueUnits=deg/s
  Rigid Transform : sm_lib/Frames and Transforms/Rigid Transform  TranslationMethod=StandardAxis  TranslationStandardOffset=0.5  TranslationLengthUnit=mm  TranslationStandardAxis=+X  TranslationCartesianOffset=[0 0 0]  TranslationROffset=0  TranslationROffsetUnits=m  TranslationZOffset=0  TranslationZOffsetUnits=m  TranslationThetaOffset=0  TranslationThetaOffsetUnits=deg  RotationMethod=None  RotationAngleUnits=deg  RotationStandardAxis=+Z  RotationAngle=0.0  RotationArbitraryAxis=[0 0 1]  FollAlignAxisA=+X  BaseAlignAxisA=+Y  FollAlignAxisB=+Y  BaseAlignAxisB=+Z  RotationSequenceAxes=FollowerAxes  RotationSequence=XYX  RotationSequenceAngles=[0 0 0]  RotationSequenceAnglesUnits=deg  RotationMatrix=[1 0 0; 0 1 0; 0 0 1]
  B : PMIOPort  Side=Right
  F : PMIOPort  Port=2  Side=Left
  connections:
  Revolute Joint1/LConn1 -- Cylindrical Solid/RConn1 -- Common Gear Constraint/LConn1
  Rigid Transform/LConn1 -- Revolute Joint1/RConn1
  Common Gear Constraint/RConn1 -- F/RConn1
  B/RConn1 -- Rigid Transform/RConn1

== system quadruped/robot enviroment/RL/leg/lower joint/joint ==
  in : Inport
  Abs1 : Abs
  Bus Creator1 : BusCreator  Inputs=4
  Bus Creator2 : BusCreator  Inputs=3
  "Hip joint " : sm_lib/Joints/Revolute Joint  JointMode=Normal  SenseConstraintForce=off  SenseConstraintForceX=off  SenseConstraintForceY=off  SenseConstraintForceZ=off  SenseConstraintTorque=off  SenseConstraintTorqueX=off  SenseConstraintTorqueY=off  SenseConstraintTorqueZ=off  SenseTotalForce=off  SenseTotalForceX=off  SenseTotalForceY=off  SenseTotalForceZ=off  SenseTotalTorque=off  SenseTotalTorqueX=off  SenseTotalTorqueY=off  SenseTotalTorqueZ=off  CompositeWrenchDir=FollowerOnBase  CompositeWrenchFrame=BaseFrame  EquilibriumPosition=0  EquilibriumPositionUnits=rad  SpringStiffness=Joint.stiffness  SpringStiffnessUnits=N*m/deg  DampingCoefficient=Joint.damping  DampingCoefficientUnits=N*m/(deg/s)  TorqueActuationMode=InputTorque  MotionActuationMode=ComputedMotion  SensePosition=on  SenseVelocity=on  SenseAcceleration=on  SenseTorqueForce=on  SenseLowerLimitTorqueForce=off  SenseUpperLimitTorqueForce=off  LowerLimitSpecify=off  LowerLimitBound=-90  LowerLimitBoundUnits=deg  LowerLimitStiffness=1e4  LowerLimitStiffnessUnits=N*m/deg  LowerLimitDamping=10  LowerLimitDampingUnits=N*m/(deg/s)  LowerLimitTransitionRegionWidth=0.1  LowerLimitTransitionRegionWidthUnits=deg  UpperLimitSpecify=off  UpperLimitBound=90  UpperLimitBoundUnits=deg  UpperLimitStiffness=1e4  UpperLimitStiffnessUnits=N*m/deg  UpperLimitDamping=10  UpperLimitDampingUnits=N*m/(deg/s)  UpperLimitTransitionRegionWidth=0.1  UpperLimitTransitionRegionWidthUnits=deg  PositionTargetSpecify=on  PositionTargetPriority=High  PositionTargetValue=Joint.base_angle  PositionTargetValueUnits=rad  VelocityTargetSpecify=off  VelocityTargetPriority=High  VelocityTargetValue=0  VelocityTargetValueUnits=deg/s
  PS-Simulink Converter{3..6} (4 alike) : nesl_utility/PS-Simulink Converter  PhysicalDomain=network_engine_domain  SubClassName=ps_output  LeftPortType=input  RightPortType=output  PseudoPeriodic=off  Frequencies=[]  Unit=inherit  AffineConversion=off
  actuator : Subsystem  mask{Actuator=Joint.actuator}
  motor inertia : Subsystem
  B : PMIOPort  Side=Left
  F : PMIOPort  Port=2  Side=Right
  p : Outport
  wires:
  PS-Simulink Converter5/1 -> Bus Creator1/3  "b"
  PS-Simulink Converter6/1 -> Abs1/1, Bus Creator1/4  "t"
  PS-Simulink Converter3/1 -> Bus Creator1/2  "w"
  in/1 -> actuator/1(in)
  Bus Creator1/1 -> actuator/2(fb)
  actuator/1(p) -> Bus Creator2/3  "actuator"
  Bus Creator2/1 -> p/1
  Abs1/1 -> Bus Creator2/2  "joint torque"
  PS-Simulink Converter4/1 -> Bus Creator2/1, Bus Creator1/1  "position"
  connections:
  "Hip joint "/RConn4 -- PS-Simulink Converter5/LConn1
  motor inertia/RConn1 -- "Hip joint "/LConn1 -- B/RConn1
  actuator/RConn1 -- "Hip joint "/LConn2
  "Hip joint "/RConn5 -- PS-Simulink Converter6/LConn1
  "Hip joint "/RConn2 -- PS-Simulink Converter4/LConn1
  "Hip joint "/RConn1 -- motor inertia/LConn1 -- F/RConn1
  "Hip joint "/RConn3 -- PS-Simulink Converter3/LConn1

== system quadruped/robot enviroment/RL/leg/upper joint/joint ==
  in : Inport
  Abs1 : Abs
  Bus Creator1 : BusCreator  Inputs=4
  Bus Creator2 : BusCreator  Inputs=3
  "Hip joint " : sm_lib/Joints/Revolute Joint  JointMode=Normal  SenseConstraintForce=off  SenseConstraintForceX=off  SenseConstraintForceY=off  SenseConstraintForceZ=off  SenseConstraintTorque=off  SenseConstraintTorqueX=off  SenseConstraintTorqueY=off  SenseConstraintTorqueZ=off  SenseTotalForce=off  SenseTotalForceX=off  SenseTotalForceY=off  SenseTotalForceZ=off  SenseTotalTorque=off  SenseTotalTorqueX=off  SenseTotalTorqueY=off  SenseTotalTorqueZ=off  CompositeWrenchDir=FollowerOnBase  CompositeWrenchFrame=BaseFrame  EquilibriumPosition=0  EquilibriumPositionUnits=rad  SpringStiffness=Joint.stiffness  SpringStiffnessUnits=N*m/deg  DampingCoefficient=Joint.damping  DampingCoefficientUnits=N*m/(deg/s)  TorqueActuationMode=InputTorque  MotionActuationMode=ComputedMotion  SensePosition=on  SenseVelocity=on  SenseAcceleration=on  SenseTorqueForce=on  SenseLowerLimitTorqueForce=off  SenseUpperLimitTorqueForce=off  LowerLimitSpecify=off  LowerLimitBound=-90  LowerLimitBoundUnits=deg  LowerLimitStiffness=1e4  LowerLimitStiffnessUnits=N*m/deg  LowerLimitDamping=10  LowerLimitDampingUnits=N*m/(deg/s)  LowerLimitTransitionRegionWidth=0.1  LowerLimitTransitionRegionWidthUnits=deg  UpperLimitSpecify=off  UpperLimitBound=90  UpperLimitBoundUnits=deg  UpperLimitStiffness=1e4  UpperLimitStiffnessUnits=N*m/deg  UpperLimitDamping=10  UpperLimitDampingUnits=N*m/(deg/s)  UpperLimitTransitionRegionWidth=0.1  UpperLimitTransitionRegionWidthUnits=deg  PositionTargetSpecify=on  PositionTargetPriority=High  PositionTargetValue=Joint.base_angle  PositionTargetValueUnits=rad  VelocityTargetSpecify=off  VelocityTargetPriority=High  VelocityTargetValue=0  VelocityTargetValueUnits=deg/s
  PS-Simulink Converter{3..6} (4 alike) : nesl_utility/PS-Simulink Converter  PhysicalDomain=network_engine_domain  SubClassName=ps_output  LeftPortType=input  RightPortType=output  PseudoPeriodic=off  Frequencies=[]  Unit=inherit  AffineConversion=off
  actuator : Subsystem  mask{Actuator=Joint.actuator}
  motor inertia : Subsystem
  B : PMIOPort  Side=Left
  F : PMIOPort  Port=2  Side=Right
  p : Outport
  wires:
  PS-Simulink Converter5/1 -> Bus Creator1/3  "b"
  PS-Simulink Converter6/1 -> Abs1/1, Bus Creator1/4  "t"
  PS-Simulink Converter3/1 -> Bus Creator1/2  "w"
  in/1 -> actuator/1(in)
  Bus Creator1/1 -> actuator/2(fb)
  actuator/1(p) -> Bus Creator2/3  "actuator"
  Bus Creator2/1 -> p/1
  Abs1/1 -> Bus Creator2/2  "joint torque"
  PS-Simulink Converter4/1 -> Bus Creator2/1, Bus Creator1/1  "position"
  connections:
  "Hip joint "/RConn4 -- PS-Simulink Converter5/LConn1
  motor inertia/RConn1 -- "Hip joint "/LConn1 -- B/RConn1
  actuator/RConn1 -- "Hip joint "/LConn2
  "Hip joint "/RConn5 -- PS-Simulink Converter6/LConn1
  "Hip joint "/RConn2 -- PS-Simulink Converter4/LConn1
  "Hip joint "/RConn1 -- motor inertia/LConn1 -- F/RConn1
  "Hip joint "/RConn3 -- PS-Simulink Converter3/LConn1

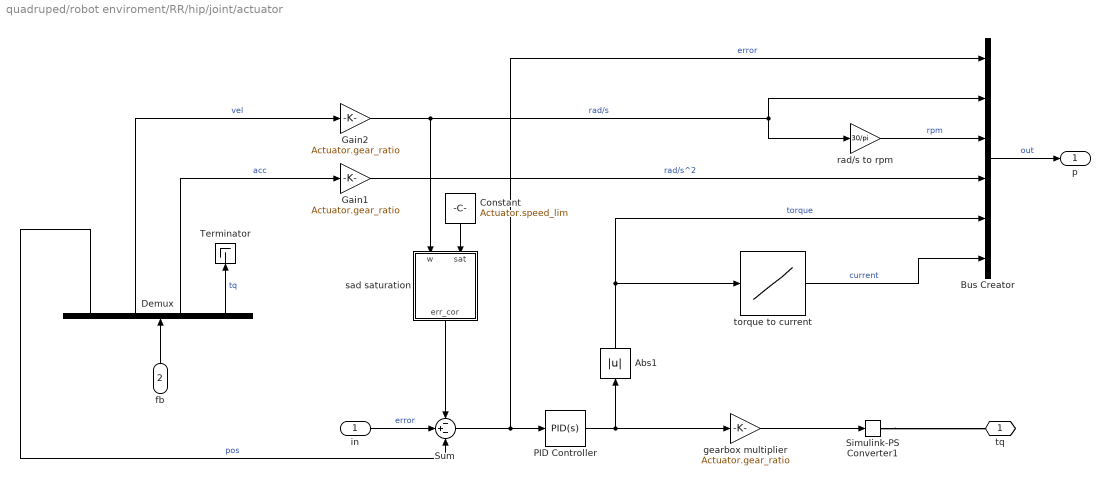
== system quadruped/robot enviroment/RR/hip/joint/actuator ==
  in : Inport
  fb : Inport  Port=2
  Abs1 : Abs
  Bus Creator : BusCreator  Inputs=6
  Constant : Constant  Value=Actuator.speed_lim
  Demux : Demux
  Gain1 : Gain  Gain=Actuator.gear_ratio
  Gain2 : Gain  Gain=Actuator.gear_ratio
  PID Controller : simulink/Continuous/PID Controller  Controller=PID  Form=Ideal  TimeDomain=Continuous-time  SampleTime=-1  IntegratorMethod=Forward Euler  FilterMethod=Forward Euler  ControllerParametersSource=internal  P=Actuator.Kp * pi / 180  I=Actuator.Ki  D=Actuator.Kd  UseFilter=on  N=Actuator.N  TunerSelectOption=Transfer Function Based (PID Tuner App)  InitialConditionSource=internal  InitialConditionForIntegrator=0  InitialConditionForFilter=0  DifferentiatorICPrevScaledInput=0  ExternalReset=none  TrackingMode=off  Kt=1  LimitOutput=on  UpperSaturationLimit=Actuator.torque_lim  LowerSaturationLimit=-Actuator.torque_lim  LinearizeAsGain=on  AntiWindupMode=none  Kb=1  POutMin=[]  POutMax=[]  IOutMin=[]  IOutMax=[]  DOutMin=[]  DOutMax=[]  NOutMin=[]  NOutMax=[]  SumOutMin=[]  SumOutMax=[]  SaturationOutMin=[]  SaturationOutMax=[]  PParamMin=[]  PParamMax=[]  IParamMin=[]  IParamMax=[]  DParamMin=[]  DParamMax=[]  NParamMin=[]  NParamMax=[]  KbParamMin=[]  KbParamMax=[]  KtParamMin=[]  KtParamMax=[]  KbOutMin=[]  KbOutMax=[]  KtOutMin=[]  KtOutMax=[]  IntegratorOutMin=[]  IntegratorOutMax=[]  FilterOutMin=[]  FilterOutMax=[]  SumI1OutMin=[]  SumI1OutMax=[]  SumI2OutMin=[]  SumI2OutMax=[]  SumI3OutMin=[]  SumI3OutMax=[]  SumI4OutMin=[]  SumI4OutMax=[]  SumDOutMin=[]  SumDOutMax=[]  DifferentiatorOutMin=[]  DifferentiatorOutMax=[]  FilterDiffOutCoefMin=[]  FilterDiffOutCoefMax=[]  ReciprocalOutMin=[]  ReciprocalOutMax=[]  SumDenOutMin=[]  SumDenOutMax=[]  SumNumOutMin=[]  SumNumOutMax=[]  DivideOutMin=[]  DivideOutMax=[]  IntegratorContinuousStateAttributes=''  IntegratorStateMustResolveToSignalObject=off  IntegratorRTWStateStorageClass=Auto  FilterContinuousStateAttributes=''  FilterStateMustResolveToSignalObject=off  FilterRTWStateStorageClass=Auto  ParallelPVariant=Passthrough  IdealPVariant=InternalParameters  IVariant=InternalParameters  DVariant=InternalParameters  IntegratorVariant=Continuous  SatVariant=Enabled  AWVariant=Passthrough  PCopyVariant=Disabled  TRVariant=Disabled  FdbkBlocksVariant=Forward  IdealPFdbkVariant=Disabled  SatFdbkVariant=Disabled  DerivativeFilterVariant=ContFilter  NVariant=InternalParameters  NCopyVariant=Disabled  FilterICVariant=InternalICsFilter  IntegratorICVariant=InternalICs  ExternalResetVariant=Disabled  TRSumVariant=Passthrough  SumFdbkVariant=Disabled  SumVariant=Sum_PID
  Simulink-PS Converter1 : nesl_utility/Simulink-PS Converter  PhysicalDomain=network_engine_domain  SubClassName=ps_input  LeftPortType=input  RightPortType=output  PseudoPeriodic=off  Frequencies=[]  NoiseDistribution=none  NoiseParameters=[]  Unit=N*m  AffineConversion=off  FilteringAndDerivatives=provide  SimscapeFilterOrder=1  InputFilterTimeConstant=0.001  UdotUserProvided=0
  Sum : Sum  Inputs=-+-
  Terminator : Terminator
  gearbox multiplier : Gain  Gain=Actuator.gear_ratio
  rad/s to rpm : Gain  Gain=30/pi
  sad saturation : Subsystem
  torque to current : Lookup_n-D  NumberOfTableDimensions=1  BreakpointsForDimension1=Actuator.torque_to_current(1,:)  Table=Actuator.torque_to_current(2,:)  InternalRulePriority=Speed  RndMeth=Simplest  InputSameDT=on
  tq : PMIOPort  Side=Right
  p : Outport
  wires:
  rad/s to rpm/1 -> Bus Creator/3  "rpm"
  Bus Creator/1 -> p/1  "out"
  torque to current/1 -> Bus Creator/6  "current"
  Sum/1 -> PID Controller/1, Bus Creator/1  "error"
  in/1 -> Sum/2  "error"
  Abs1/1 -> Bus Creator/5, torque to current/1  "torque"
  PID Controller/1 -> gearbox multiplier/1, Abs1/1
  gearbox multiplier/1 -> Simulink-PS Converter1/1
  Gain2/1 -> rad/s to rpm/1, Bus Creator/2, sad saturation/1(w)  "rad/s"
  fb/1 -> Demux/1
  Demux/1 -> Sum/3  "pos"
  Demux/2 -> Gain2/1  "vel"
  Demux/3 -> Gain1/1  "acc"
  Demux/4 -> Terminator/1  "tq"
  Gain1/1 -> Bus Creator/4  "rad/s^2"
  sad saturation/1(err_cor) -> Sum/1
  Constant/1 -> sad saturation/2(sat)
  connections:
  Simulink-PS Converter1/RConn1 -- tq/RConn1
